simulink model "LQR"  (R2025b)
settings: Solver=VariableStepAuto  StartTime=0.0  StopTime=10.0  RelTol=1e-3
values from neighbouring files (symbols this model uses):
  A = [ 0     1        0 ... (first row only)    [compare.m]    (also in compute_lqr_gains.m = [ 0    1      0)
  B = [0; 0; 1/Lc]    [compare.m]    (also in compute_lqr_gains.m)
  C = eye(3)    [compare.m]
  D = zeros(3,1)    [compare.m]
  K = [Ko(1) Ko(2) Ki]    [compute_lqr_gains.m]
settings Model: PacingRate=4

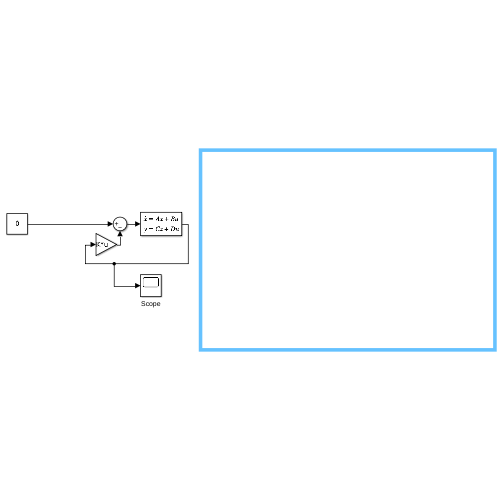
[thumbnail: Simulink's stored preview of the top-level diagram]
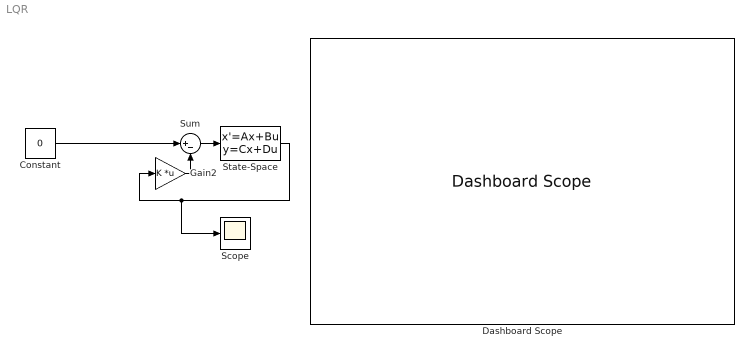
== system LQR ==
  Constant : Constant  Value=0
  Dashboard Scope : DashboardScope  FontColor=[0.0, 0.0, 0.0]
  Gain2 : Gain  Gain=K  Multiplication=Matrix(K*u)
  Scope : Scope
      settings: ActiveDisplayYMinimum=-0.026259170738630138  ActiveDisplayYMaximum=0.027144657722210478
  State-Space : StateSpace  A=A  B=B  C=C  D=D  InitialCondition=[0.1,0,0]  ContinuousStateAttributes='pos'
  Sum : Sum  Inputs=|+-
  wires:
  Constant/1 -> Sum/1
  Gain2/1 -> Sum/2
  State-Space/1 -> Scope/1, Gain2/1
  Sum/1 -> State-Space/1
